simulink model "Cruise_control"  (R2020b)
settings: Solver=ode45  StartTime=0.0  StopTime=120  RelTol=1e-3
values from neighbouring files (symbols this model uses):
  b = 50    [Init.m]    (also in prob3_Cruise_Control.sldd = 50.0)
  Ki = 150    [Init.m]    (also in prob3_Cruise_Control.sldd = 200.0)
  Kp = 80    [Init.m]    (also in prob3_Cruise_Control.sldd = 400.0)
  m = 1000    [Init.m]    (also in prob3_Cruise_Control.sldd = 1000.0)
  Ts = 0.01    [Init.m]    (also in prob3_Cruise_Control.sldd)
settings Model: Creator=Rasika Shejul  LastModifiedBy=Rasika Shejul

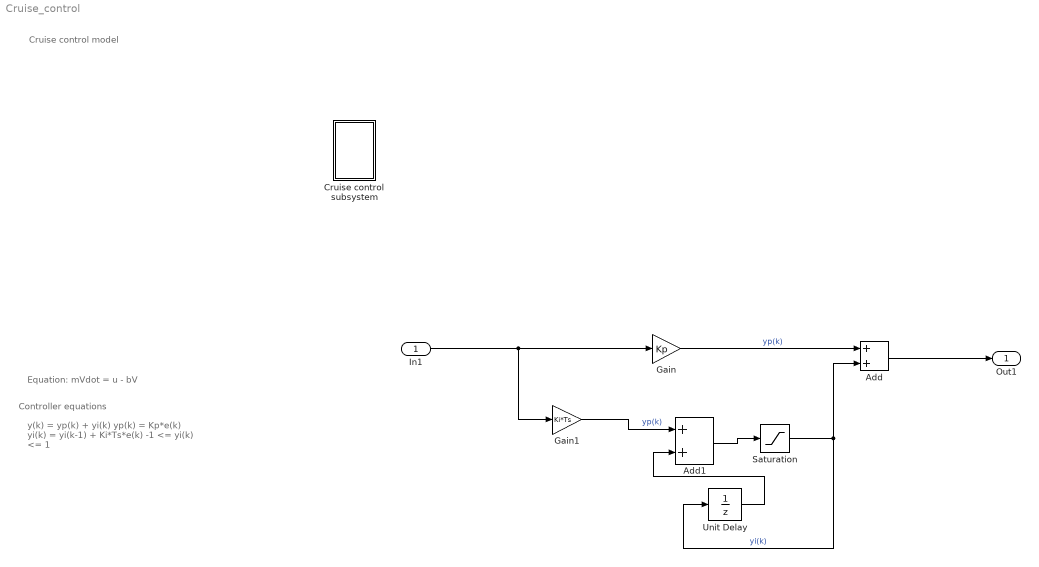
== system Cruise_control ==
  note: Controller equations
  note: y(k) = yp(k) + yi(k)
      | yp(k) = Kp*e(k)
      | yi(k) = yi(k-1) + Ki*Ts*e(k)
      | -1 <= yi(k) <= 1
  note: Equation:
      | mVdot = u - bV
  note: Cruise control model
  In1 : Inport
  Add : Sum
  Add1 : Sum
  Cruise control subsystem : Subsystem
  Gain : Gain  Gain=Kp
  Gain1 : Gain  Gain=Ki*Ts
  Saturation : Saturate  UpperLimit=1  LowerLimit=-1
  Unit Delay : UnitDelay  SampleTime=-1  HasFrameUpgradeWarning=on
  Out1 : Outport
  wires:
  Gain1/1 -> Add1/1  "yp(k)"
  Add1/1 -> Saturation/1
  Saturation/1 -> Add/2, Unit Delay/1  "yi(k)"
  Add/1 -> Out1/1
  Gain/1 -> Add/1  "yp(k)"
  In1/1 -> Gain1/1, Gain/1
  Unit Delay/1 -> Add1/2

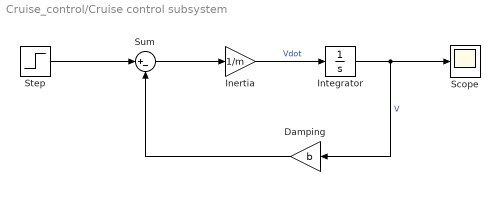
== system Cruise_control/Cruise control subsystem ==
  Damping : Gain  Gain=b
  Inertia : Gain  Gain=1/m
  Integrator : Integrator
  Scope : Scope
  Step : Step  After=u  SampleTime=0
  Sum : Sum  Inputs=|+-
  wires:
  Step/1 -> Sum/1
  Inertia/1 -> Integrator/1  "Vdot"
  Integrator/1 -> Damping/1, Scope/1  "V"
  Damping/1 -> Sum/2
  Sum/1 -> Inertia/1
